simulink subsystem "Gyroscope"  (R2021a)
settings: Solver=VariableStepAuto  StartTime=0.0  StopTime=10.0  RelTol=1e-3
undefined symbols (not defined in the file): sensors, Ts
libraries: simulink x4, dspsrcs4 x3
settings Model: Creator=Laura  LastModifiedBy=Laura

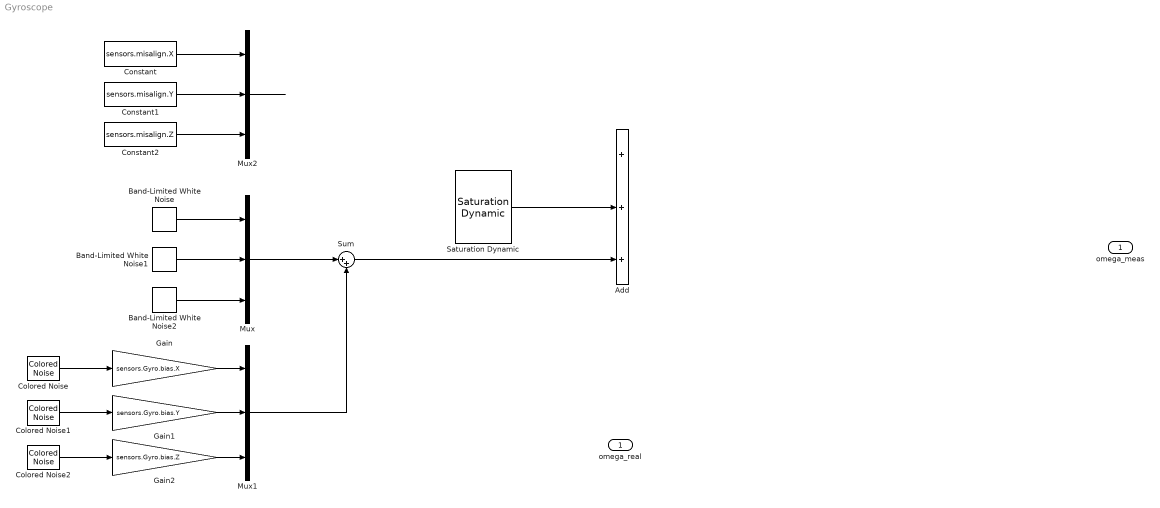
== system Gyroscope ==
  omega_real : Inport
  Add : Sum  Inputs=+++
  Band-Limited White Noise : simulink/Sources/Band-Limited White Noise  Cov=sensors.gyro.NoisePower.X  Ts=Ts  seed=[23341]
  Band-Limited White Noise1 : simulink/Sources/Band-Limited White Noise  Cov=sensors.gyro.NoisePower.Y  Ts=Ts  seed=[23341]
  Band-Limited White Noise2 : simulink/Sources/Band-Limited White Noise  Cov=sensors.gyro.NoisePower.Z  Ts=Ts  seed=[23341]
  Colored Noise : dspsrcs4/Colored Noise  Color=pink  InverseFrequencyPower=1  BoundedOutput=off  NumChannels=1  OutputDataType=double  SamplesPerFrame=1  SampleTime=Ts  RandomStream=mt19937ar with seed  Seed=67  SimulateUsing=Interpreted execution
      settings: SourceProductBaseCode=DS
  Colored Noise1 : dspsrcs4/Colored Noise  Color=pink  InverseFrequencyPower=1  BoundedOutput=off  NumChannels=1  OutputDataType=double  SamplesPerFrame=1  SampleTime=Ts  RandomStream=mt19937ar with seed  Seed=67  SimulateUsing=Interpreted execution
      settings: SourceProductBaseCode=DS
  Colored Noise2 : dspsrcs4/Colored Noise  Color=pink  InverseFrequencyPower=1  BoundedOutput=off  NumChannels=1  OutputDataType=double  SamplesPerFrame=1  SampleTime=Ts  RandomStream=mt19937ar with seed  Seed=67  SimulateUsing=Interpreted execution
      settings: SourceProductBaseCode=DS
  Constant : Constant  Value=sensors.misalign.X
  Constant1 : Constant  Value=sensors.misalign.Y
  Constant2 : Constant  Value=sensors.misalign.Z
  Gain : Gain  Gain=sensors.Gyro.bias.X
  Gain1 : Gain  Gain=sensors.Gyro.bias.Y
  Gain2 : Gain  Gain=sensors.Gyro.bias.Z
  Mux : Mux  Inputs=3
  Mux1 : Mux  Inputs=3
  Mux2 : Mux  Inputs=3
  Saturation Dynamic : simulink/Discontinuities/Saturation Dynamic  OutMin=[]  OutMax=[]  OutDataTypeStr=Inherit: Same as second input  OutDataType=fixdt(1, 16)  OutScaling=2^-10  DoSatur=off
  Sum : Sum  Inputs=|++
  omega_meas : Outport
  wires:
  Band-Limited White Noise2/1 -> Mux/3
  Band-Limited White Noise1/1 -> Mux/2
  Band-Limited White Noise/1 -> Mux/1
  Mux/1 -> Sum/1
  Saturation Dynamic/1 -> Add/2
  Colored Noise/1 -> Gain/1
  Gain/1 -> Mux1/1
  Colored Noise1/1 -> Gain1/1
  Gain1/1 -> Mux1/2
  Colored Noise2/1 -> Gain2/1
  Gain2/1 -> Mux1/3
  Mux1/1 -> Sum/2
  Sum/1 -> Add/3
  Constant1/1 -> Mux2/2
  Constant/1 -> Mux2/1
  Constant2/1 -> Mux2/3
  Mux2/1 -> ?
